simulink model "ThdRwRtStCaller"  (R2018b)
settings: Solver=FixedStepDiscrete  StartTime=0.0  StopTime=10.0  RelTol=1e-3
undefined symbols (not defined in the file or in its folder): ThdRwRtStBkReclnCtrl_1_Cal, ThdRwRtStBkReclnHolderChk_1_Cal, ThdRwRtStBkReclnIsPosChk_1_Cal, ThdRwRtStCshnFldCtrl_1_Cal, ThdRwRtStCshnFldHolderChk_1_Cal, ThdRwRtStCshnFldIsPosChk_1_Cal, ThdRwRtStFwdBkwdCtrl_1_Cal, ThdRwRtStFwdBkwdHolderChk_1_Cal, ThdRwRtStFwdBkwdIsPosChk_1_Cal, ThdRwRtStFwdBkwdSpdCtrl_1_Cal, ThdRwRtStRclCmdSrvCal_1_Cal, ThrdRwRtStBkReclnTrgtPosSelc_1_Cal, ThrdRwRtStCshnFldTrgtPosSelc_1_Cal, ThrdRwRtStFwdBkwdTrgtPosSelc_1_Cal
settings Model: Creator=sn2xws  LastModifiedBy=sn2xws
settings DataIOCC: SaveFormat=StructureWithTime
settings OptimizationCC: DefaultParameterBehavior=Inlined  EnhancedBackFolding=on  PassReuseOutputArgsAs=Individual arguments  ZeroExternalMemoryAtStartup=off  ZeroInternalMemoryAtStartup=off  OptimizeBlockOrder=speed  DifferentSizesBufferReuse=on  OptimizationCustomize=off
settings DebuggingCC: ParameterTunabilityLossMsg=error
settings SFSimCC: MATLABDynamicMemAlloc=off
settings RTWCC: SystemTargetFile=autosar.tlc  GenCodeOnly=on  TemplateMakefile=ert_default_tmf  Description=AUTOSAR  GenerateReport=on  IncludeHyperlinkInReport=on  LaunchReport=on  GenerateTraceInfo=on  GenerateTraceReport=on  GenerateTraceReportSl=on  GenerateTraceReportSf=on  GenerateTraceReportEml=on
settings CodeAppCC: ForceParamTrailComments=on  IgnoreCustomStorageClasses=off  OperatorAnnotations=on  SimulinkDataObjDesc=on  SFDataObjDesc=on  InsertBlockDesc=on
settings STFCustomTargetCC: TargetLangStandard=C99 (ISO)  MultiwordLength=256  ParMdlRefBuildCompliant=on  CompOptLevelCompliant=on  IncludeMdlTerminateFcn=off  CombineOutputUpdateFcns=on  SuppressErrorStatus=on  ERTCustomFileBanners=on  SupportNonFinite=off  SupportComplex=off  SupportContinuousTime=off  SupportNonInlinedSFcns=off  RemoveResetFunc=on  MATLABClassNameForMDSCustomization=Simulink.SoftwareTarget.ERTCustomization  AutosarCompliant=on  UseToolchainInfoCompliant=on  LookupTableObjectStructAxisOrder=2,1,3,4,...  LUTObjectStructOrderEvenSpacing=Size,Table,Breakpoints  SystemTargetFile=autosar.tlc
settings ERTTargetCC: TargetLangStandard=C99 (ISO)  ConcurrentExecutionCompliant=off  IncludeMdlTerminateFcn=off  SuppressErrorStatus=on  SupportNonFinite=off  SupportComplex=off  ModelStepFunctionPrototypeControlCompliant=off  CPPClassGenCompliant=off  AutosarCompliant=on  LookupTableObjectStructAxisOrder=2,1,3,4,...  LUTObjectStructOrderEvenSpacing=Size,Table,Breakpoints  InlinedParameterPlacement=NonHierarchical  ERTCustomFileTemplate=example_file_process.tlc  ERTFilePackagingFormat=Compact

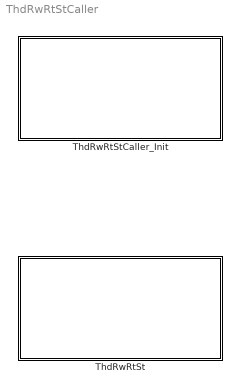
== system ThdRwRtStCaller ==
  ThdRwRtSt : Subsystem
  ThdRwRtStCaller_Init : Subsystem

== system ThdRwRtStCaller/ThdRwRtSt ==
  ThdRwRtSt_Cal_sys : Subsystem

== system ThdRwRtStCaller/ThdRwRtStCaller_Init ==
  Event Listener : EventListener  EventName=reset

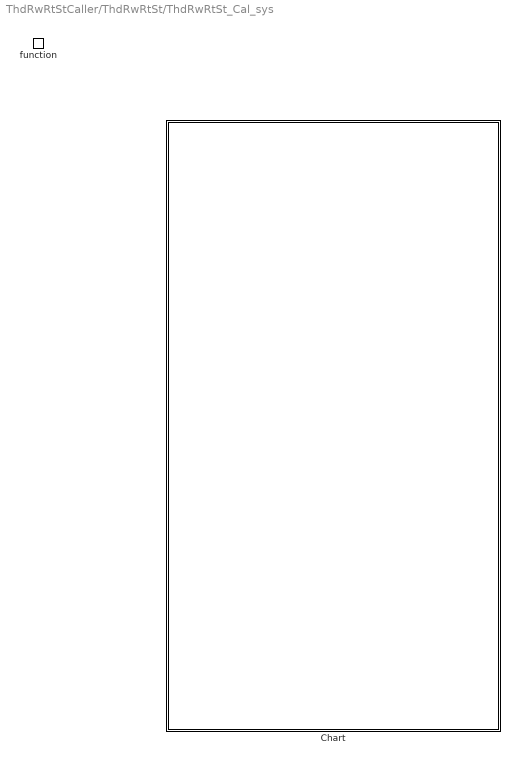
== system ThdRwRtStCaller/ThdRwRtSt/ThdRwRtSt_Cal_sys ==
  function : TriggerPort  TriggerType=function-call  IsSimulinkFunction=on  FunctionName=ThdRwRtSt_Cal  VariantControl=(inherit)
  Chart : Stateflow chart  TreatAsAtomicUnit=on

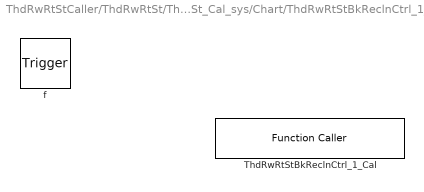
== system ThdRwRtStCaller/ThdRwRtSt/ThdRwRtSt_Cal_sys/Chart/ThdRwRtStBkReclnCtrl_1_Cal ==
  f : TriggerPort  TriggerType=function-call  VariantControl=(inherit)
      settings: CopyFcn=Stateflow.SLINSF.SimulinkMan.removeBlockPreDeleteFcn  PreDeleteFcn=Stateflow.SLINSF.SimulinkMan.unsafePredeleteFcn
  ThdRwRtStBkReclnCtrl_1_Cal : FunctionCaller  FunctionPrototype=ThdRwRtStBkReclnCtrl_1_Cal()

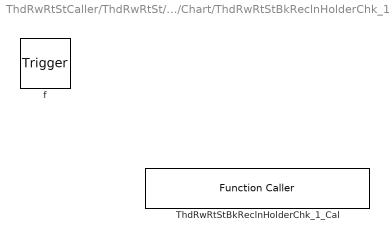
== system ThdRwRtStCaller/ThdRwRtSt/ThdRwRtSt_Cal_sys/Chart/ThdRwRtStBkReclnHolderChk_1_Cal ==
  f : TriggerPort  TriggerType=function-call  VariantControl=(inherit)
      settings: CopyFcn=Stateflow.SLINSF.SimulinkMan.removeBlockPreDeleteFcn  PreDeleteFcn=Stateflow.SLINSF.SimulinkMan.unsafePredeleteFcn
  ThdRwRtStBkReclnHolderChk_1_Cal : FunctionCaller  FunctionPrototype=ThdRwRtStBkReclnHolderChk_1_Cal()

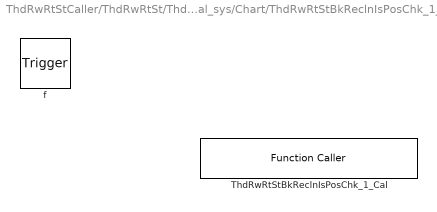
== system ThdRwRtStCaller/ThdRwRtSt/ThdRwRtSt_Cal_sys/Chart/ThdRwRtStBkReclnIsPosChk_1_Cal ==
  f : TriggerPort  TriggerType=function-call  VariantControl=(inherit)
      settings: CopyFcn=Stateflow.SLINSF.SimulinkMan.removeBlockPreDeleteFcn  PreDeleteFcn=Stateflow.SLINSF.SimulinkMan.unsafePredeleteFcn
  ThdRwRtStBkReclnIsPosChk_1_Cal : FunctionCaller  FunctionPrototype=ThdRwRtStBkReclnIsPosChk_1_Cal()

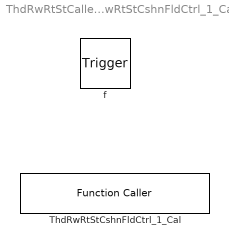
== system ThdRwRtStCaller/ThdRwRtSt/ThdRwRtSt_Cal_sys/Chart/ThdRwRtStCshnFldCtrl_1_Cal ==
  f : TriggerPort  TriggerType=function-call  VariantControl=(inherit)
      settings: CopyFcn=Stateflow.SLINSF.SimulinkMan.removeBlockPreDeleteFcn  PreDeleteFcn=Stateflow.SLINSF.SimulinkMan.unsafePredeleteFcn
  ThdRwRtStCshnFldCtrl_1_Cal : FunctionCaller  FunctionPrototype=ThdRwRtStCshnFldCtrl_1_Cal()

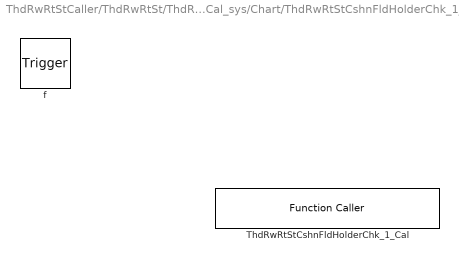
== system ThdRwRtStCaller/ThdRwRtSt/ThdRwRtSt_Cal_sys/Chart/ThdRwRtStCshnFldHolderChk_1_Cal ==
  f : TriggerPort  TriggerType=function-call  VariantControl=(inherit)
      settings: CopyFcn=Stateflow.SLINSF.SimulinkMan.removeBlockPreDeleteFcn  PreDeleteFcn=Stateflow.SLINSF.SimulinkMan.unsafePredeleteFcn
  ThdRwRtStCshnFldHolderChk_1_Cal : FunctionCaller  FunctionPrototype=ThdRwRtStCshnFldHolderChk_1_Cal()

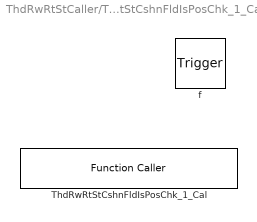
== system ThdRwRtStCaller/ThdRwRtSt/ThdRwRtSt_Cal_sys/Chart/ThdRwRtStCshnFldIsPosChk_1_Cal ==
  f : TriggerPort  TriggerType=function-call  VariantControl=(inherit)
      settings: CopyFcn=Stateflow.SLINSF.SimulinkMan.removeBlockPreDeleteFcn  PreDeleteFcn=Stateflow.SLINSF.SimulinkMan.unsafePredeleteFcn
  ThdRwRtStCshnFldIsPosChk_1_Cal : FunctionCaller  FunctionPrototype=ThdRwRtStCshnFldIsPosChk_1_Cal()

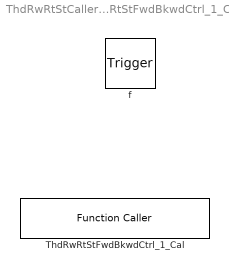
== system ThdRwRtStCaller/ThdRwRtSt/ThdRwRtSt_Cal_sys/Chart/ThdRwRtStFwdBkwdCtrl_1_Cal ==
  f : TriggerPort  TriggerType=function-call  VariantControl=(inherit)
      settings: CopyFcn=Stateflow.SLINSF.SimulinkMan.removeBlockPreDeleteFcn  PreDeleteFcn=Stateflow.SLINSF.SimulinkMan.unsafePredeleteFcn
  ThdRwRtStFwdBkwdCtrl_1_Cal : FunctionCaller  FunctionPrototype=ThdRwRtStFwdBkwdCtrl_1_Cal()

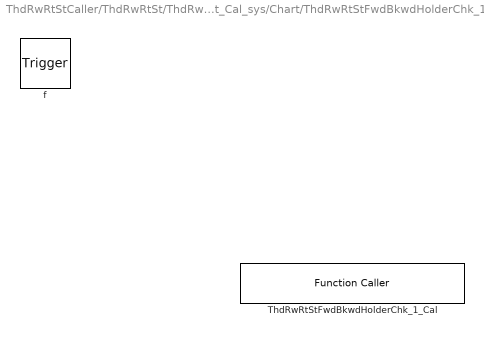
== system ThdRwRtStCaller/ThdRwRtSt/ThdRwRtSt_Cal_sys/Chart/ThdRwRtStFwdBkwdHolderChk_1_Cal ==
  f : TriggerPort  TriggerType=function-call  VariantControl=(inherit)
      settings: CopyFcn=Stateflow.SLINSF.SimulinkMan.removeBlockPreDeleteFcn  PreDeleteFcn=Stateflow.SLINSF.SimulinkMan.unsafePredeleteFcn
  ThdRwRtStFwdBkwdHolderChk_1_Cal : FunctionCaller  FunctionPrototype=ThdRwRtStFwdBkwdHolderChk_1_Cal()

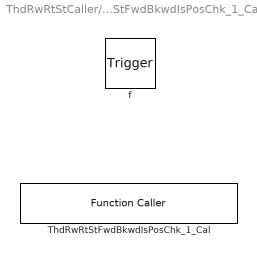
== system ThdRwRtStCaller/ThdRwRtSt/ThdRwRtSt_Cal_sys/Chart/ThdRwRtStFwdBkwdIsPosChk_1_Cal ==
  f : TriggerPort  TriggerType=function-call  VariantControl=(inherit)
      settings: CopyFcn=Stateflow.SLINSF.SimulinkMan.removeBlockPreDeleteFcn  PreDeleteFcn=Stateflow.SLINSF.SimulinkMan.unsafePredeleteFcn
  ThdRwRtStFwdBkwdIsPosChk_1_Cal : FunctionCaller  FunctionPrototype=ThdRwRtStFwdBkwdIsPosChk_1_Cal()

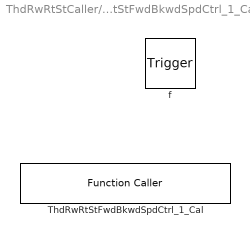
== system ThdRwRtStCaller/ThdRwRtSt/ThdRwRtSt_Cal_sys/Chart/ThdRwRtStFwdBkwdSpdCtrl_1_Cal ==
  f : TriggerPort  TriggerType=function-call  VariantControl=(inherit)
      settings: CopyFcn=Stateflow.SLINSF.SimulinkMan.removeBlockPreDeleteFcn  PreDeleteFcn=Stateflow.SLINSF.SimulinkMan.unsafePredeleteFcn
  ThdRwRtStFwdBkwdSpdCtrl_1_Cal : FunctionCaller  FunctionPrototype=ThdRwRtStFwdBkwdSpdCtrl_1_Cal()

== system ThdRwRtStCaller/ThdRwRtSt/ThdRwRtSt_Cal_sys/Chart/ThdRwRtStRclCmdSrvCal_1_Cal ==
  f : TriggerPort  TriggerType=function-call  VariantControl=(inherit)
      settings: CopyFcn=Stateflow.SLINSF.SimulinkMan.removeBlockPreDeleteFcn  PreDeleteFcn=Stateflow.SLINSF.SimulinkMan.unsafePredeleteFcn
  ThdRwRtStRclCmdSrvCal_1_Cal : FunctionCaller  FunctionPrototype=ThdRwRtStRclCmdSrvCal_1_Cal()

== system ThdRwRtStCaller/ThdRwRtSt/ThdRwRtSt_Cal_sys/Chart/ThrdRwRtStBkReclnTrgtPosSelc_1_Cal ==
  f : TriggerPort  TriggerType=function-call  VariantControl=(inherit)
      settings: CopyFcn=Stateflow.SLINSF.SimulinkMan.removeBlockPreDeleteFcn  PreDeleteFcn=Stateflow.SLINSF.SimulinkMan.unsafePredeleteFcn
  ThrdRwRtStBkReclnTrgtPosSelc_1_Cal : FunctionCaller  FunctionPrototype=ThrdRwRtStBkReclnTrgtPosSelc_1_Cal()

== system ThdRwRtStCaller/ThdRwRtSt/ThdRwRtSt_Cal_sys/Chart/ThrdRwRtStCshnFldTrgtPosSelc_1_Cal ==
  f : TriggerPort  TriggerType=function-call  VariantControl=(inherit)
      settings: CopyFcn=Stateflow.SLINSF.SimulinkMan.removeBlockPreDeleteFcn  PreDeleteFcn=Stateflow.SLINSF.SimulinkMan.unsafePredeleteFcn
  ThrdRwRtStCshnFldTrgtPosSelc_1_Cal : FunctionCaller  FunctionPrototype=ThrdRwRtStCshnFldTrgtPosSelc_1_Cal()

== system ThdRwRtStCaller/ThdRwRtSt/ThdRwRtSt_Cal_sys/Chart/ThrdRwRtStFwdBkwdTrgtPosSelc_1_Cal ==
  f : TriggerPort  TriggerType=function-call  VariantControl=(inherit)
      settings: CopyFcn=Stateflow.SLINSF.SimulinkMan.removeBlockPreDeleteFcn  PreDeleteFcn=Stateflow.SLINSF.SimulinkMan.unsafePredeleteFcn
  ThrdRwRtStFwdBkwdTrgtPosSelc_1_Cal : FunctionCaller  FunctionPrototype=ThrdRwRtStFwdBkwdTrgtPosSelc_1_Cal()

== stateflow chart ThdRwRtStCaller/ThdRwRtSt/ThdRwRtSt_Cal_sys/Chart ==
  state ThrdRwRtStBkReclnTrgtPosSelc_1_Cal [function]
  state ThrdRwRtStCshnFldTrgtPosSelc_1_Cal [function]
  state ThrdRwRtStFwdBkwdTrgtPosSelc_1_Cal [function]
  state ThdRwRtStBkReclnHolderChk_1_Cal [function]
  state ThdRwRtStCshnFldHolderChk_1_Cal [function]
  state ThdRwRtStFwdBkwdHolderChk_1_Cal [function]
  state ThdRwRtStBkReclnIsPosChk_1_Cal [function]
  state ThdRwRtStCshnFldIsPosChk_1_Cal [function]
  state ThdRwRtStFwdBkwdIsPosChk_1_Cal [function]
  state ThdRwRtStBkReclnCtrl_1_Cal [function]
  state ThdRwRtStCshnFldCtrl_1_Cal [function]
  state ThdRwRtStFwdBkwdCtrl_1_Cal [function]
  state ThdRwRtStFwdBkwdSpdCtrl_1_Cal [function]
  state ThdRwRtStRclCmdSrvCal_1_Cal [function]
  (default) -> (junction 15)
  (junction 15) -> (junction 17) : {
      | ThrdRwRtStBkReclnTrgtPosSelc_1_Cal();
      | ThrdRwRtStCshnFldTrgtPosSelc_1_Cal();
      | ThrdRwRtStFwdBkwdTrgtPosSelc_1_Cal();
      | ThdRwRtStBkReclnIsPosChk_1_Cal();
      | ThdRwRtStCshnFldIsPosChk_1_Cal();
      | ThdRwRtStFwdBkwdIsPosChk_1_Cal();
      | ThdRwRtStBkReclnHolderChk_1_Cal();
      | ThdRwRtStCshnFldHolderChk_1_Cal();
      | ThdRwRtStFwdBkwdHolderChk_1_Cal();
      | ThdRwRtStBkReclnCtrl_1_Cal();
      | ThdRwRtStCshnFldCtrl_1_Cal();
      | ThdRwRtStFwdBkwdCtrl_1_Cal();
      | ThdRwRtStFwdBkwdSpdCtrl_1_Cal();
      | ThdRwRtStRclCmdSrvCal_1_Cal();
      | }
